simulink model "tf_cooling_water"  (R2020a)
settings: Solver=FixedStepAuto  StartTime=0.0  StopTime=10.0  RelTol=1e-3
model workspace (MAT data in the model file):
  ambient_temp = 25
  mcp_max_cooling_water_temp = 90
  tau = 50
undefined symbols (not defined in the file): mcp_nominal_rotation
settings Model: OrderedModelArguments=off  Creator=Luiz  LastModifiedBy=ToT_IPMS_03

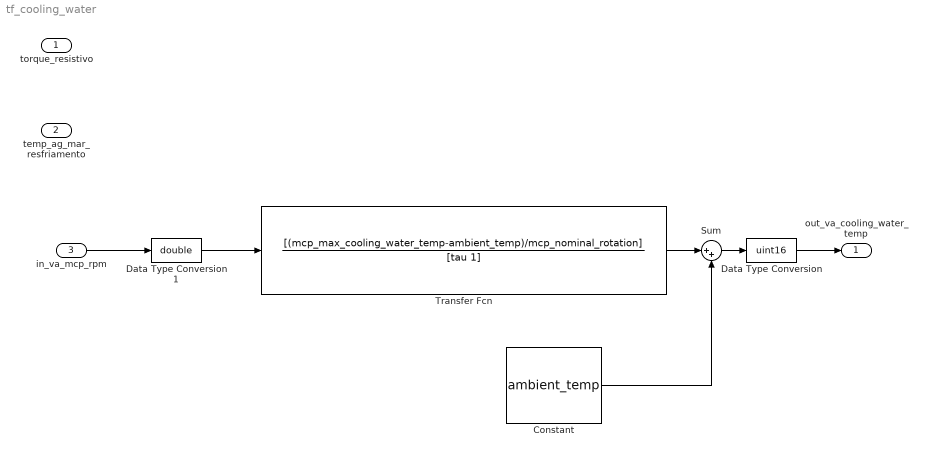
== system tf_cooling_water ==
  torque_resistivo : Inport  OutDataTypeStr=double
  temp_ag_mar_resfriamento : Inport  Port=2  OutDataTypeStr=uint16
  in_va_mcp_rpm : Inport  Port=3  OutMin=[0]  OutMax=[mcp_nominal_rotation]  OutDataTypeStr=uint16  Unit=rpm  LockScale=on
  Constant : Constant  Value=ambient_temp
  Data Type Conversion : DataTypeConversion  OutDataTypeStr=uint16
  Data Type Conversion1 : DataTypeConversion  OutDataTypeStr=double
  Sum : Sum  Inputs=|++
  Transfer Fcn : TransferFcn  Numerator=[(mcp_max_cooling_water_temp-ambient_temp)/mcp_nominal_rotation]  Denominator=[tau 1]
  out_va_cooling_water_temp : Outport  OutMin=[0]  OutMax=[90]  OutDataTypeStr=uint16  Unit=°C
  wires:
  Transfer Fcn/1 -> Sum/1
  Constant/1 -> Sum/2
  in_va_mcp_rpm/1 -> Data Type Conversion1/1
  Sum/1 -> Data Type Conversion/1
  Data Type Conversion/1 -> out_va_cooling_water_temp/1
  Data Type Conversion1/1 -> Transfer Fcn/1
